simulink model "model_a29"  (R2020a)
settings: Solver=FixedStepAuto  StartTime=0.0  StopTime=10  FixedStep=0.001  RelTol=1e-3
undefined symbols (not defined in the file or in its folder): DiscIntNeverNeededParam
settings Model: Creator=Daniel  LastModifiedBy=Daniel

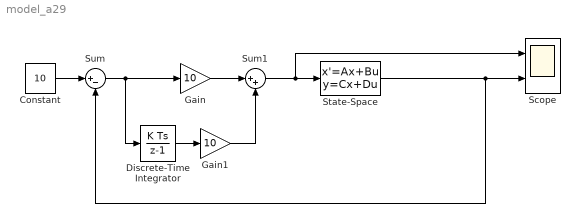
== system model_a29 ==
  Constant : Constant  Value=10
  Discrete-Time Integrator : DiscreteIntegrator  SampleTime=-1  ICPrevOutput=DiscIntNeverNeededParam  ICPrevScaledInput=DiscIntNeverNeededParam
  Gain : Gain  Gain=10
  Gain1 : Gain  Gain=10
  Scope : Scope  NumInputPorts=2
  State-Space : StateSpace  A=-1  D=0  InitialCondition=0
  Sum : Sum  Inputs=|+-
  Sum1 : Sum  Inputs=|++
  wires:
  Constant/1 -> Sum/1
  Sum/1 -> Discrete-Time Integrator/1, Gain/1
  State-Space/1 -> Scope/2, Sum/2
  Gain/1 -> Sum1/1
  Sum1/1 -> Scope/1, State-Space/1
  Discrete-Time Integrator/1 -> Gain1/1
  Gain1/1 -> Sum1/2
